simulink model "FCTCR"  (R2025a)
settings: Solver=VariableStepAuto  StartTime=0.0  StopTime=1  RelTol=1e-3
undefined symbols (not defined in the file): a
libraries: spsVoltageMeasurementLib x4, spsCurrentMeasurementLib x3, spsSeriesRLCBranchLib x3, spsThyristorLib x2, spsACVoltageSourceLib x1, sps_lib x1
settings Model: Creator=prajw  LastModifiedBy=Subu Aryal

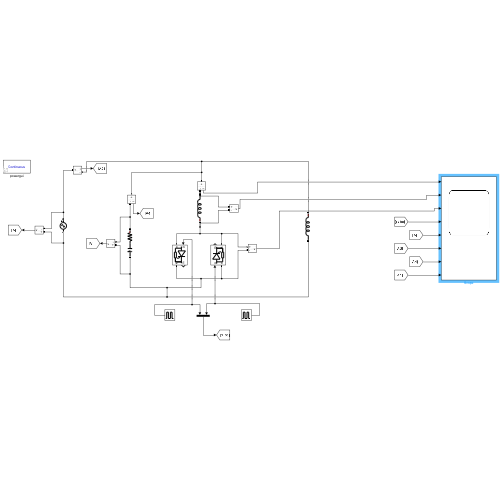
[thumbnail: Simulink's stored preview of the top-level diagram]
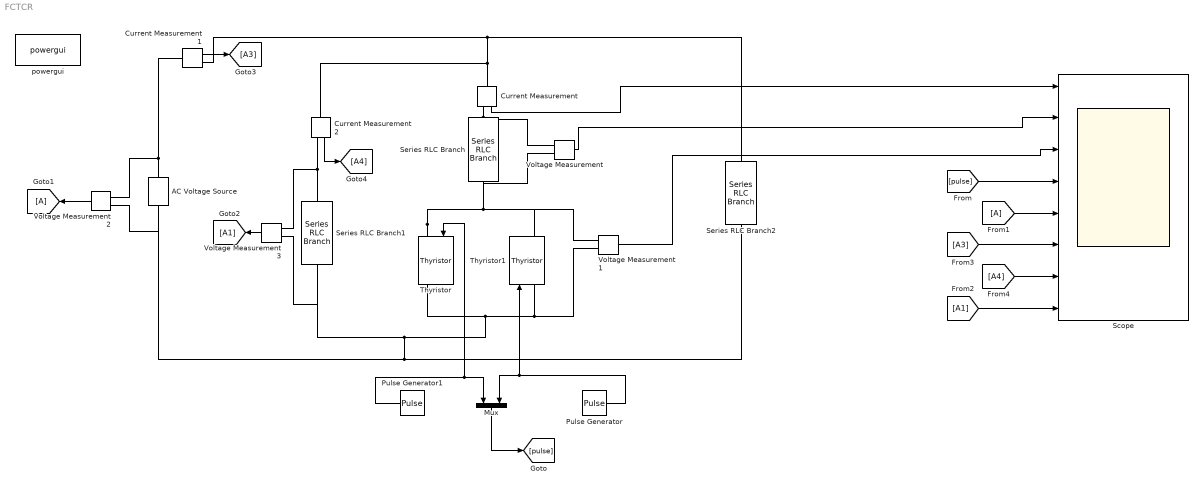
== system FCTCR ==
  AC Voltage Source : spsACVoltageSourceLib/AC Voltage Source  Amplitude=100  Phase=0  Frequency=50  SampleTime=0  Measurements=None  BusType=swing  Pref=10e3  Qref=0  Qmin=-inf  Qmax=+inf
  Current Measurement : spsCurrentMeasurementLib/Current Measurement  PhasorSimulation=off  OutputType=Complex  PSBequivalent=0
  Current Measurement1 : spsCurrentMeasurementLib/Current Measurement  PhasorSimulation=off  OutputType=Complex  PSBequivalent=0
  Current Measurement2 : spsCurrentMeasurementLib/Current Measurement  PhasorSimulation=off  OutputType=Complex  PSBequivalent=0
  From1 : From
  Goto1 : Goto
  Mux : Mux  Inputs=2
  Pulse Generator : DiscretePulseGenerator  PulseType=Time based  Period=1/50  PulseWidth=0.1  PhaseDelay=((0.02/360)*(a+180))
  Pulse Generator1 : DiscretePulseGenerator  PulseType=Time based  Period=1/50  PulseWidth=0.1  PhaseDelay=((0.02/360)*a)
  Scope : Scope  NumInputPorts=8
      settings: Title=Inductor Current  ActiveDisplayYMinimum=-0.019622043625254514  ActiveDisplayYMaximum=0.019622142055509093  YLabel=IL
  Series RLC Branch : spsSeriesRLCBranchLib/Series RLC Branch  LConnTagsString=__new0  RConnTagsString=__new0  BranchType=L  Resistance=1  Inductance=1e-3  SetiL0=off  InitialCurrent=0  Capacitance=1e-6  Setx0=off  InitialVoltage=0  Measurements=None
  Series RLC Branch1 : spsSeriesRLCBranchLib/Series RLC Branch  LConnTagsString=__new0  RConnTagsString=__new0  BranchType=RC  Resistance=0.001  Inductance=1e-3  SetiL0=off  InitialCurrent=0  Capacitance=10e-3  Setx0=off  InitialVoltage=0  Measurements=None
  Series RLC Branch2 : spsSeriesRLCBranchLib/Series RLC Branch  LConnTagsString=__new0  RConnTagsString=__new0  BranchType=L  Resistance=0.01  Inductance=1e-3  SetiL0=off  InitialCurrent=0  Capacitance=1e-6  Setx0=off  InitialVoltage=0  Measurements=None
  Thyristor : spsThyristorLib/Thyristor  Ron=0.001  Lon=0  Vf=0.8  IC=0  Rs=500  Cs=250e-9  Measurements=on
  Thyristor1 : spsThyristorLib/Thyristor  Ron=0.001  Lon=0  Vf=0.8  IC=0  Rs=500  Cs=250e-9  Measurements=on
  Voltage Measurement{,1..3} (4 alike) : spsVoltageMeasurementLib/Voltage Measurement  PhasorSimulation=off  OutputType=Complex  PSBequivalent=0
  powergui : sps_lib/powergui  Priority=1  SimulationMode=Continuous  SampleTime=50e-6  frequency=60  Iterations=50  frequencyindice=50  Pbase=100e6  ErrMax=1e-4  UnitsV=kV  UnitsW=MW  buscounter=0  FunctionMessages=off  echomessages=off  EnableUseOfTLC=off  CurrentSourceSwitches=off  DisableSnubberDevices=off  DisableRonSwitches=off  DisableVfSwitches=off  DisplayEquations=off  AutomaticDiscreteSolvers=off  SolverType=Tustin/Backward Euler (TBE)  Interpol=off  ExternalGateDelay=off  methode=off  Ts=100  x0status=blocks  SPID=on  SwTol=0  HookPort=off  NonlinearTolerance=1e-4  nMaxIteration=100  ContinueOnMaxIteration=off  RestoreLinks=warning  ResistiveCurrentMeasurement=off  Frange=[0:2:500]  Ylog=off  Xlog=on  ShowGrid=off  save=off  variable=ZData  structure=0  ZoomFFT=off  StartTime=0.0  cycles=1  DisplayStyle=1  fundamental=60  FreqAxis=off  MaxFrequency=1000  frequencyindicesteady=1  RmsSteady=1  display=off
  wires:
  Voltage Measurement/1 -> Scope/2
  [pulse] -> Scope/4
  From1/1 -> Scope/5
  Mux/1 -> [pulse]
  Voltage Measurement2/1 -> Goto1/1
  Pulse Generator/1 -> Mux/2, Thyristor1/1
  Current Measurement/1 -> Scope/1
  Voltage Measurement1/1 -> Scope/3
  Pulse Generator1/1 -> Mux/1, Thyristor/1
  Voltage Measurement3/1 -> [A1]
  [A1] -> Scope/8
  Current Measurement1/1 -> [A3]
  [A3] -> Scope/6
  Current Measurement2/1 -> [A4]
  [A4] -> Scope/7
  connections:
  Voltage Measurement3/LConn2 -- Series RLC Branch1/LConn1 -- Current Measurement2/RConn1
  Thyristor/LConn1 -- Series RLC Branch/LConn1 -- Voltage Measurement/LConn2 -- Voltage Measurement1/LConn1 -- Thyristor1/RConn1
  Series RLC Branch2/LConn1 -- Current Measurement2/LConn1 -- Current Measurement/LConn1 -- Current Measurement1/RConn1
  Voltage Measurement1/LConn2 -- Voltage Measurement3/LConn1 -- Series RLC Branch1/RConn1 -- Series RLC Branch2/RConn1 -- AC Voltage Source/LConn1 -- Voltage Measurement2/LConn1 -- Thyristor/RConn1 -- Thyristor1/LConn1
  Voltage Measurement2/LConn2 -- AC Voltage Source/RConn1 -- Current Measurement1/LConn1
  Current Measurement/RConn1 -- Series RLC Branch/RConn1 -- Voltage Measurement/LConn1
